simulink model "untitled"  (R2022b)
settings: Solver=VariableStepAuto  StartTime=0.0  StopTime=3  MaxStep=1e-3  RelTol=1e-3
model workspace (MAT data in the model file):
  x0 = 0
undefined symbols (not defined in the file or in its folder): x_0
settings Model: Creator=21.00127-8  LastModifiedBy=21.00127-8

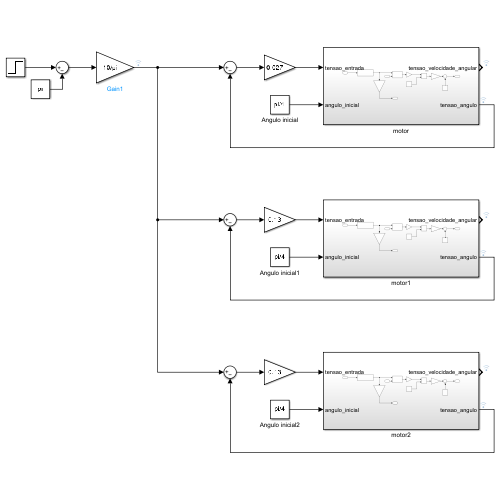
[thumbnail: Simulink's stored preview of the top-level diagram]
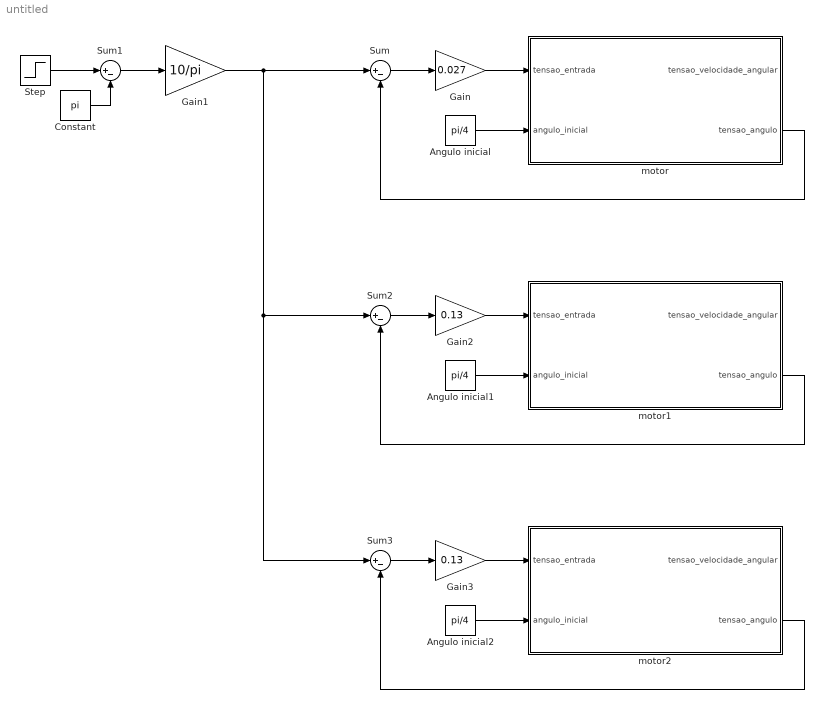
== system untitled ==
  Angulo inicial : Constant  Value=pi/4
  Angulo inicial1 : Constant  Value=pi/4
  Angulo inicial2 : Constant  Value=pi/4
  Constant : Constant  Value=pi
  Gain : Gain  Gain=0.027
  Gain1 : Gain  Gain=10/pi
  Gain2 : Gain  Gain=0.13
  Gain3 : Gain  Gain=0.13
  Step : Step  Before=pi/4  After=pi/2  SampleTime=0
  Sum{,1..3} (4 alike) : Sum  Inputs=|+-
  motor : Subsystem
  motor1 : Subsystem
  motor2 : Subsystem
  wires:
  Angulo inicial/1 -> motor/2(angulo_inicial)
  Gain/1 -> motor/1(tensao_entrada)
  Sum/1 -> Gain/1
  motor/2(tensao_angulo) -> Sum/2
  Step/1 -> Sum1/1
  Sum1/1 -> Gain1/1
  Constant/1 -> Sum1/2
  motor1/2(tensao_angulo) -> Sum2/2
  Sum2/1 -> Gain2/1
  Gain2/1 -> motor1/1(tensao_entrada)
  Angulo inicial1/1 -> motor1/2(angulo_inicial)
  Angulo inicial2/1 -> motor2/2(angulo_inicial)
  Gain3/1 -> motor2/1(tensao_entrada)
  Sum3/1 -> Gain3/1
  motor2/2(tensao_angulo) -> Sum3/2
  Gain1/1 -> Sum3/1, Sum2/1, Sum/1

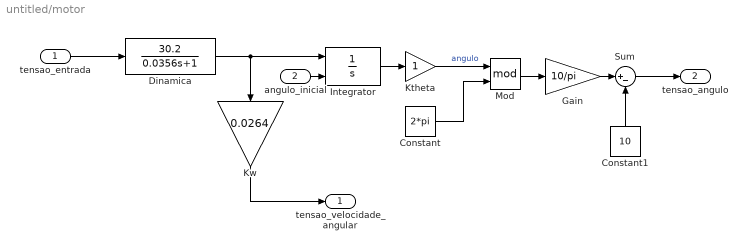
== system untitled/motor ==
  tensao_entrada : Inport
  angulo_inicial : Inport  Port=2
  Constant : Constant  Value=2*pi
  Constant1 : Constant  Value=10
  Dinamica : TransferFcn  Numerator=[30.2]  Denominator=[0.0356 1]
  Gain : Gain  Gain=10/pi
  Integrator : Integrator  InitialConditionSource=external  InitialCondition=x_0
  Ktheta : Gain
  Kw : Gain  Gain=0.0264
  Mod : Math  Operator=mod
  Sum : Sum  Inputs=|+-
  tensao_velocidade_angular : Outport
  tensao_angulo : Outport  Port=2
  wires:
  Dinamica/1 -> Integrator/1, Kw/1
  tensao_entrada/1 -> Dinamica/1
  Integrator/1 -> Ktheta/1
  Kw/1 -> tensao_velocidade_angular/1
  Ktheta/1 -> Mod/1  "angulo"
  Constant/1 -> Mod/2
  Mod/1 -> Gain/1
  Gain/1 -> Sum/1
  Constant1/1 -> Sum/2
  Sum/1 -> tensao_angulo/1
  angulo_inicial/1 -> Integrator/2

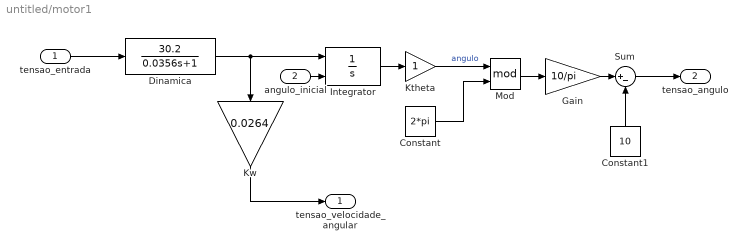
== system untitled/motor1 ==
  tensao_entrada : Inport
  angulo_inicial : Inport  Port=2
  Constant : Constant  Value=2*pi
  Constant1 : Constant  Value=10
  Dinamica : TransferFcn  Numerator=[30.2]  Denominator=[0.0356 1]
  Gain : Gain  Gain=10/pi
  Integrator : Integrator  InitialConditionSource=external  InitialCondition=x_0
  Ktheta : Gain
  Kw : Gain  Gain=0.0264
  Mod : Math  Operator=mod
  Sum : Sum  Inputs=|+-
  tensao_velocidade_angular : Outport
  tensao_angulo : Outport  Port=2
  wires:
  angulo_inicial/1 -> Integrator/2
  Sum/1 -> tensao_angulo/1
  Constant1/1 -> Sum/2
  Gain/1 -> Sum/1
  Mod/1 -> Gain/1
  Constant/1 -> Mod/2
  Ktheta/1 -> Mod/1  "angulo"
  Kw/1 -> tensao_velocidade_angular/1
  Integrator/1 -> Ktheta/1
  tensao_entrada/1 -> Dinamica/1
  Dinamica/1 -> Kw/1, Integrator/1

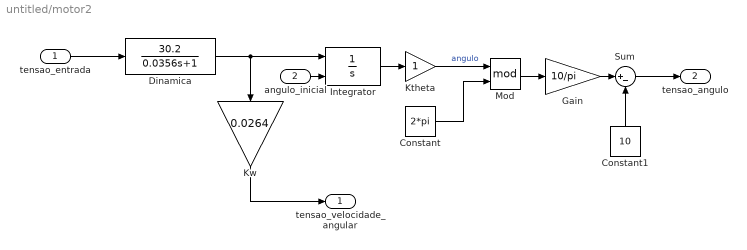
== system untitled/motor2 ==
  tensao_entrada : Inport
  angulo_inicial : Inport  Port=2
  Constant : Constant  Value=2*pi
  Constant1 : Constant  Value=10
  Dinamica : TransferFcn  Numerator=[30.2]  Denominator=[0.0356 1]
  Gain : Gain  Gain=10/pi
  Integrator : Integrator  InitialConditionSource=external  InitialCondition=x_0
  Ktheta : Gain
  Kw : Gain  Gain=0.0264
  Mod : Math  Operator=mod
  Sum : Sum  Inputs=|+-
  tensao_velocidade_angular : Outport
  tensao_angulo : Outport  Port=2
  wires:
  Dinamica/1 -> Integrator/1, Kw/1
  tensao_entrada/1 -> Dinamica/1
  Integrator/1 -> Ktheta/1
  Kw/1 -> tensao_velocidade_angular/1
  Ktheta/1 -> Mod/1  "angulo"
  Constant/1 -> Mod/2
  Mod/1 -> Gain/1
  Gain/1 -> Sum/1
  Constant1/1 -> Sum/2
  Sum/1 -> tensao_angulo/1
  angulo_inicial/1 -> Integrator/2
